simulink model "ThreeL_PWM_direct_2018b"  (R2018b)
settings: Solver=VariableStepAuto  StartTime=0.0  StopTime=0.05  RelTol=1e-3
InitFcn:
  | f_pwm_clk=100e6;
  | T_pwm_clk=1/f_pwm_clk;
libraries: hdlsllib x1
settings Model: Creator=BHK  LastModifiedBy=ga92wum
settings OptimizationCC: BlockReduction=off  ConditionallyExecuteInputs=off  DefaultParameterBehavior=Inlined
settings DebuggingCC: AlgebraicLoopMsg=error
settings HardwareCC: ProdBitPerPointer=32  ProdBitPerSizeT=32  ProdBitPerPtrDiffT=32  ProdLargestAtomicFloat=None  ProdIntDivRoundTo=Undefined  ProdEndianess=Unspecified  ProdWordSize=32  ProdHWDeviceType=ASIC/FPGA->ASIC/FPGA  TargetBitPerPointer=64  TargetBitPerSizeT=64  TargetBitPerPtrDiffT=64  TargetLongLongMode=on  TargetIntDivRoundTo=Zero  TargetEndianess=LittleEndian  TargetWordSize=64  TargetHWDeviceType=Custom Processor->MATLAB Host Computer  ProdEqTarget=off
settings SFSimCC: SimUseLocalCustomCode=off
settings RTWCC: RTWUseLocalCustomCode=off

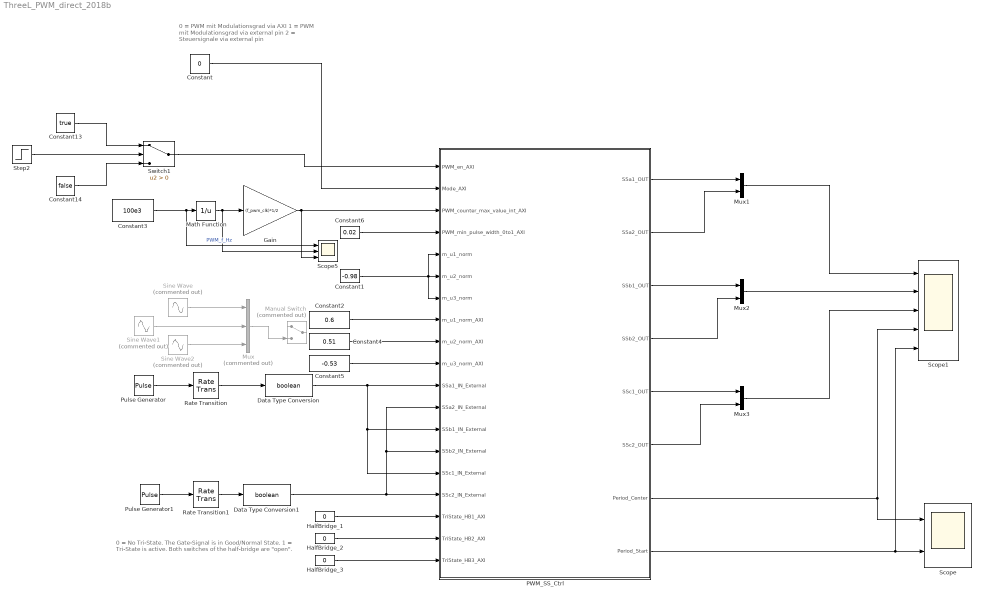
== system ThreeL_PWM_direct_2018b ==
  note: 0 = PWM mit Modulationsgrad via AXI
      | 1 = PWM mit Modulationsgrad via external pin
      | 2 = Steuersignale via external pin
  note: 0 = No Tri-State. The Gate-Signal is in Good/Normal State.
      | 1 = Tri-State is active. Both switches of the half-bridge are "open".
  Constant : Constant  Value=0  OutDataTypeStr=fixdt(0,2,0)  SampleTime=T_pwm_clk
  Constant1 : Constant  Value=-0.98  OutDataTypeStr=fixdt(1,14,12)  SampleTime=T_pwm_clk
  Constant13 : Constant  Value=true  SampleTime=T_pwm_clk
  Constant14 : Constant  Value=false  SampleTime=T_pwm_clk
  Constant2 : Constant  Value=0.6  OutDataTypeStr=fixdt(1,14,12)  SampleTime=T_pwm_clk
  Constant3 : Constant  Value=100e3  OutDataTypeStr=double  SampleTime=T_pwm_clk
  Constant4 : Constant  Value=0.51  OutDataTypeStr=fixdt(1,14,12)  SampleTime=T_pwm_clk
  Constant5 : Constant  Value=-0.53  OutDataTypeStr=fixdt(1,14,12)  SampleTime=T_pwm_clk
  Constant6 : Constant  Value=0.02  OutDataTypeStr=fixdt(1,14,12)  SampleTime=T_pwm_clk
  Data Type Conversion : DataTypeConversion  OutDataTypeStr=boolean
  Data Type Conversion1 : DataTypeConversion  OutDataTypeStr=boolean
  Gain : Gain  Gain=(f_pwm_clk)*1/2  OutDataTypeStr=fixdt(0,20,0)
  HalfBridge_1 : Constant  Value=0  OutDataTypeStr=fixdt(0,2,0)  SampleTime=T_pwm_clk
  HalfBridge_2 : Constant  Value=0  OutDataTypeStr=fixdt(0,2,0)  SampleTime=T_pwm_clk
  HalfBridge_3 : Constant  Value=0  OutDataTypeStr=fixdt(0,2,0)  SampleTime=T_pwm_clk
  Manual Switch : ManualSwitch  Commented=on
  Math Function : Math  Operator=reciprocal  SaturateOnIntegerOverflow=on
  Mux : Mux  Commented=on  Inputs=3
  Mux1 : Mux  Inputs=2
  Mux2 : Mux  Inputs=2
  Mux3 : Mux  Inputs=2
  PWM_SS_Ctrl : Subsystem  TreatAsAtomicUnit=on
  Pulse Generator : DiscretePulseGenerator  PulseType=Time based  Period=2.8e-5  PulseWidth=50  PhaseDelay=0.002
  Pulse Generator1 : DiscretePulseGenerator  PulseType=Time based  Period=2.8e-5  PulseWidth=50  PhaseDelay=0.002
  Rate Transition : RateTransition  OutPortSampleTime=T_pwm_clk
  Rate Transition1 : RateTransition  OutPortSampleTime=T_pwm_clk
  Scope : Scope  NumInputPorts=2
  Scope1 : Scope  NumInputPorts=5
  Scope5 : Scope  NumInputPorts=3
  Sine Wave : Sin  Commented=on  Amplitude=0.8  Frequency=100*pi  Phase=-0.2*pi  SampleTime=T_pwm_clk
  Sine Wave1 : Sin  Commented=on  Amplitude=0.8  Frequency=100*pi  Phase=-0.2*pi + 2/3 * pi  SampleTime=T_pwm_clk
  Sine Wave2 : Sin  Commented=on  Amplitude=0.8  Frequency=100*pi + 4/3 * pi  Phase=-0.2*pi  SampleTime=T_pwm_clk
  Step2 : Step  Time=0.002  SampleTime=T_pwm_clk
  Switch1 : Switch  Criteria=u2 > Threshold
  wires:
  Step2/1 -> Switch1/2
  Constant13/1 -> Switch1/1
  Constant14/1 -> Switch1/3
  Switch1/1 -> PWM_SS_Ctrl/1(PWM_en_AXI)
  Constant/1 -> PWM_SS_Ctrl/2(Mode_AXI)
  Constant6/1 -> PWM_SS_Ctrl/4(PWM_min_pulse_width_0to1_AXI)
  Constant1/1 -> PWM_SS_Ctrl/6(m_u2_norm), PWM_SS_Ctrl/5(m_u1_norm), PWM_SS_Ctrl/7(m_u3_norm)
  Constant3/1 -> Scope5/1, Math Function/1  "PWM_f_Hz"
  Rate Transition/1 -> Data Type Conversion/1
  Pulse Generator/1 -> Rate Transition/1
  HalfBridge_3/1 -> PWM_SS_Ctrl/19(TriState_HB3_AXI)
  HalfBridge_2/1 -> PWM_SS_Ctrl/18(TriState_HB2_AXI)
  HalfBridge_1/1 -> PWM_SS_Ctrl/17(TriState_HB1_AXI)
  Constant2/1 -> PWM_SS_Ctrl/8(m_u1_norm_AXI)
  Mux/1 -> Manual Switch/2
  Sine Wave/1 -> Mux/1
  Sine Wave1/1 -> Mux/2
  Sine Wave2/1 -> Mux/3
  PWM_SS_Ctrl/7(Period_Center) -> Scope1/4, Scope/1
  PWM_SS_Ctrl/8(Period_Start) -> Scope1/5, Scope/2
  Data Type Conversion/1 -> PWM_SS_Ctrl/13(SSb1_IN_External), PWM_SS_Ctrl/15(SSc1_IN_External), PWM_SS_Ctrl/11(SSa1_IN_External)
  Pulse Generator1/1 -> Rate Transition1/1
  Constant4/1 -> PWM_SS_Ctrl/9(m_u2_norm_AXI)
  Constant5/1 -> PWM_SS_Ctrl/10(m_u3_norm_AXI)
  Rate Transition1/1 -> Data Type Conversion1/1
  Data Type Conversion1/1 -> PWM_SS_Ctrl/14(SSb2_IN_External), PWM_SS_Ctrl/12(SSa2_IN_External), PWM_SS_Ctrl/16(SSc2_IN_External)
  PWM_SS_Ctrl/1(SSa1_OUT) -> Mux1/1
  PWM_SS_Ctrl/2(SSa2_OUT) -> Mux1/2
  Mux1/1 -> Scope1/1
  Mux2/1 -> Scope1/2
  PWM_SS_Ctrl/3(SSb1_OUT) -> Mux2/1
  PWM_SS_Ctrl/4(SSb2_OUT) -> Mux2/2
  Mux3/1 -> Scope1/3
  PWM_SS_Ctrl/5(SSc1_OUT) -> Mux3/1
  PWM_SS_Ctrl/6(SSc2_OUT) -> Mux3/2
  Gain/1 -> PWM_SS_Ctrl/3(PWM_counter_max_value_int_AXI), Scope5/3
  Math Function/1 -> Scope5/2, Gain/1

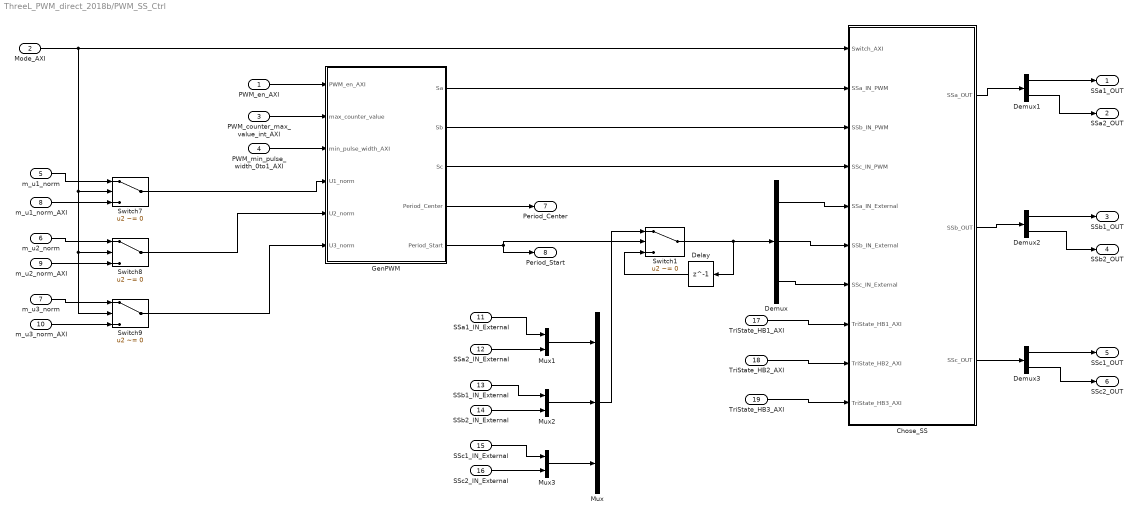
== system ThreeL_PWM_direct_2018b/PWM_SS_Ctrl ==
  PWM_en_AXI : Inport
  Mode_AXI : Inport  Port=2
  PWM_counter_max_value_int_AXI : Inport  Port=3
  PWM_min_pulse_width_0to1_AXI : Inport  Port=4
  m_u1_norm : Inport  Port=5
  m_u2_norm : Inport  Port=6
  m_u3_norm : Inport  Port=7
  m_u1_norm_AXI : Inport  Port=8
  m_u2_norm_AXI : Inport  Port=9
  m_u3_norm_AXI : Inport  Port=10
  SSa1_IN_External : Inport  Port=11
  SSa2_IN_External : Inport  Port=12
  SSb1_IN_External : Inport  Port=13
  SSb2_IN_External : Inport  Port=14
  SSc1_IN_External : Inport  Port=15
  SSc2_IN_External : Inport  Port=16
  TriState_HB1_AXI : Inport  Port=17
  TriState_HB2_AXI : Inport  Port=18
  TriState_HB3_AXI : Inport  Port=19
  Chose_SS : Subsystem
  Delay : Delay  DelayLength=1
  Demux : Demux  Outputs=3
  Demux1 : Demux  Outputs=2
  Demux2 : Demux  Outputs=2
  Demux3 : Demux  Outputs=2
  GenPWM : Subsystem  TreatAsAtomicUnit=on
  Mux : Mux  Inputs=3
  Mux1 : Mux  Inputs=2
  Mux2 : Mux  Inputs=2
  Mux3 : Mux  Inputs=2
  Switch{1,7..9} (4 alike) : Switch  Criteria=u2 ~= 0
  SSa1_OUT : Outport  VectorParamsAs1DForOutWhenUnconnected=off
  SSa2_OUT : Outport  Port=2  VectorParamsAs1DForOutWhenUnconnected=off
  SSb1_OUT : Outport  Port=3  VectorParamsAs1DForOutWhenUnconnected=off
  SSb2_OUT : Outport  Port=4  VectorParamsAs1DForOutWhenUnconnected=off
  SSc1_OUT : Outport  Port=5  VectorParamsAs1DForOutWhenUnconnected=off
  SSc2_OUT : Outport  Port=6  VectorParamsAs1DForOutWhenUnconnected=off
  Period_Center : Outport  Port=7  VectorParamsAs1DForOutWhenUnconnected=off
  Period_Start : Outport  Port=8  VectorParamsAs1DForOutWhenUnconnected=off
  wires:
  PWM_en_AXI/1 -> GenPWM/1(PWM_en_AXI)
  PWM_min_pulse_width_0to1_AXI/1 -> GenPWM/3(min_pulse_width_AXI)
  Switch9/1 -> GenPWM/6(U3_norm)
  m_u1_norm_AXI/1 -> Switch7/3
  m_u1_norm/1 -> Switch7/1
  m_u2_norm/1 -> Switch8/1
  m_u2_norm_AXI/1 -> Switch8/3
  m_u3_norm/1 -> Switch9/1
  m_u3_norm_AXI/1 -> Switch9/3
  Switch8/1 -> GenPWM/5(U2_norm)
  Switch7/1 -> GenPWM/4(U1_norm)
  PWM_counter_max_value_int_AXI/1 -> GenPWM/2(max_counter_value)
  TriState_HB1_AXI/1 -> Chose_SS/8(TriState_HB1_AXI)
  TriState_HB2_AXI/1 -> Chose_SS/9(TriState_HB2_AXI)
  TriState_HB3_AXI/1 -> Chose_SS/10(TriState_HB3_AXI)
  GenPWM/1(Sa) -> Chose_SS/2(SSa_IN_PWM)
  GenPWM/2(Sb) -> Chose_SS/3(SSb_IN_PWM)
  GenPWM/3(Sc) -> Chose_SS/4(SSc_IN_PWM)
  Mode_AXI/1 -> Switch9/2, Switch8/2, Switch7/2, Chose_SS/1(Switch_AXI)
  GenPWM/4(Period_Center) -> Period_Center/1
  Switch1/1 -> Delay/1, Demux/1
  GenPWM/5(Period_Start) -> Switch1/2, Period_Start/1
  Delay/1 -> Switch1/3
  Mux/1 -> Switch1/1
  Demux/1 -> Chose_SS/5(SSa_IN_External)
  Demux/2 -> Chose_SS/6(SSb_IN_External)
  Demux/3 -> Chose_SS/7(SSc_IN_External)
  SSa2_IN_External/1 -> Mux1/2
  SSa1_IN_External/1 -> Mux1/1
  Mux1/1 -> Mux/1
  Mux2/1 -> Mux/2
  SSb1_IN_External/1 -> Mux2/1
  SSb2_IN_External/1 -> Mux2/2
  Mux3/1 -> Mux/3
  SSc1_IN_External/1 -> Mux3/1
  SSc2_IN_External/1 -> Mux3/2
  Chose_SS/1(SSa_OUT) -> Demux1/1
  Chose_SS/2(SSb_OUT) -> Demux2/1
  Chose_SS/3(SSc_OUT) -> Demux3/1
  Demux1/1 -> SSa1_OUT/1
  Demux1/2 -> SSa2_OUT/1
  Demux2/1 -> SSb1_OUT/1
  Demux2/2 -> SSb2_OUT/1
  Demux3/1 -> SSc1_OUT/1
  Demux3/2 -> SSc2_OUT/1

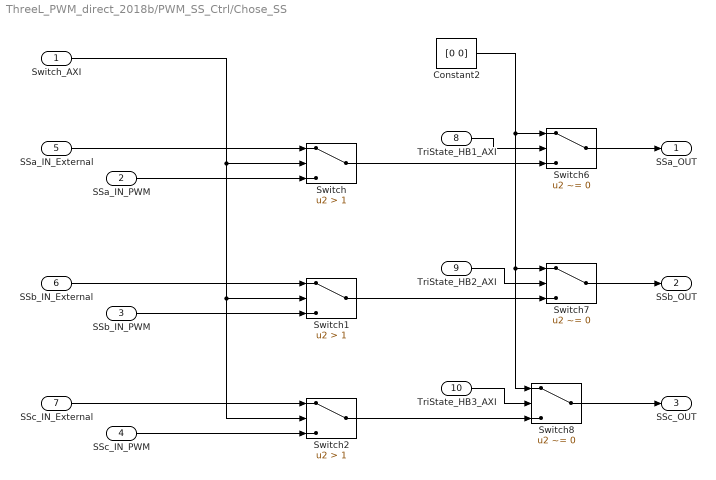
== system ThreeL_PWM_direct_2018b/PWM_SS_Ctrl/Chose_SS ==
  Switch_AXI : Inport
  SSa_IN_PWM : Inport  Port=2
  SSb_IN_PWM : Inport  Port=3
  SSc_IN_PWM : Inport  Port=4
  SSa_IN_External : Inport  Port=5
  SSb_IN_External : Inport  Port=6
  SSc_IN_External : Inport  Port=7
  TriState_HB1_AXI : Inport  Port=8
  TriState_HB2_AXI : Inport  Port=9
  TriState_HB3_AXI : Inport  Port=10
  Constant2 : Constant  Value=[0 0]  OutDataTypeStr=fixdt(0,1,0)  SampleTime=T_pwm_clk
  Switch : Switch  Criteria=u2 > Threshold  Threshold=1
  Switch1 : Switch  Criteria=u2 > Threshold  Threshold=1
  Switch2 : Switch  Criteria=u2 > Threshold  Threshold=1
  Switch6 : Switch  Criteria=u2 ~= 0  Threshold=1
  Switch7 : Switch  Criteria=u2 ~= 0  Threshold=1
  Switch8 : Switch  Criteria=u2 ~= 0  Threshold=1
  SSa_OUT : Outport  VectorParamsAs1DForOutWhenUnconnected=off
  SSb_OUT : Outport  Port=2  VectorParamsAs1DForOutWhenUnconnected=off
  SSc_OUT : Outport  Port=3  VectorParamsAs1DForOutWhenUnconnected=off
  wires:
  Switch_AXI/1 -> Switch2/2, Switch1/2, Switch/2
  Switch/1 -> Switch6/3
  Switch2/1 -> Switch8/3
  Switch1/1 -> Switch7/3
  TriState_HB2_AXI/1 -> Switch7/2
  TriState_HB1_AXI/1 -> Switch6/2
  Constant2/1 -> Switch8/1, Switch7/1, Switch6/1
  SSa_IN_PWM/1 -> Switch/3
  SSb_IN_PWM/1 -> Switch1/3
  SSc_IN_PWM/1 -> Switch2/3
  SSb_IN_External/1 -> Switch1/1
  SSc_IN_External/1 -> Switch2/1
  SSa_IN_External/1 -> Switch/1
  TriState_HB3_AXI/1 -> Switch8/2
  Switch6/1 -> SSa_OUT/1
  Switch7/1 -> SSb_OUT/1
  Switch8/1 -> SSc_OUT/1

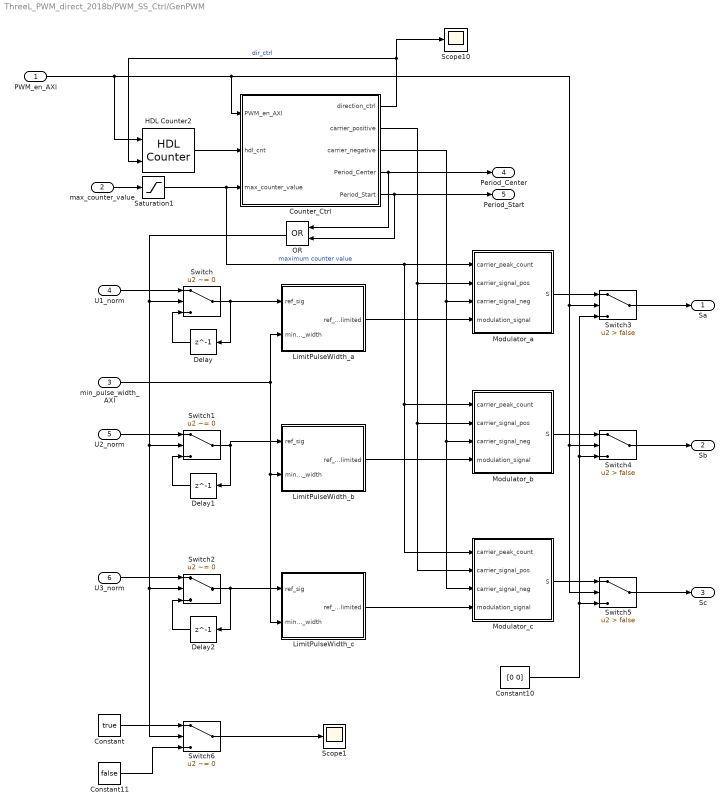
== system ThreeL_PWM_direct_2018b/PWM_SS_Ctrl/GenPWM ==
  PWM_en_AXI : Inport
  max_counter_value : Inport  Port=2
  min_pulse_width_AXI : Inport  Port=3
  U1_norm : Inport  Port=4
  U2_norm : Inport  Port=5
  U3_norm : Inport  Port=6
  Constant : Constant  Value=true  SampleTime=T_pwm_clk
  Constant10 : Constant  Value=[0 0]  OutDataTypeStr=fixdt(0,1,0)  SampleTime=T_pwm_clk
  Constant11 : Constant  Value=false  SampleTime=T_pwm_clk
  Counter_Ctrl : Subsystem
  Delay : Delay  DelayLength=1
  Delay1 : Delay  DelayLength=1
  Delay2 : Delay  DelayLength=1
  HDL Counter2 : hdlsllib/Sources/HDL Counter  CountType=Free running  CountInit=0  CountStep=1  CountMax=100  CountFromType=Initial value  CountFrom=0  CountResetPort=off  CountLoadPort=off  CountEnbPort=on  CountDirPort=on  CountDataType=Unsigned  CountWordLen=20  CountFracLen=0  CountSampTime=1
      settings: SourceProductBaseCode=HD
  LimitPulseWidth_a : Subsystem
  LimitPulseWidth_b : Subsystem
  LimitPulseWidth_c : Subsystem
  Modulator_a : Subsystem
  Modulator_b : Subsystem
  Modulator_c : Subsystem
  OR : Logic  Operator=OR  AllPortsSameDT=off  OutDataTypeStr=boolean
  Saturation1 : Saturate  UpperLimit=10000*50  LowerLimit=10*50
  Scope1 : Scope
  Scope10 : Scope
  Switch{,1..2,6} (4 alike) : Switch  Criteria=u2 ~= 0
  Switch3 : Switch  Criteria=u2 > Threshold  Threshold=false
  Switch4 : Switch  Criteria=u2 > Threshold  Threshold=false
  Switch5 : Switch  Criteria=u2 > Threshold  Threshold=false
  Sa : Outport  VectorParamsAs1DForOutWhenUnconnected=off
  Sb : Outport  Port=2  VectorParamsAs1DForOutWhenUnconnected=off
  Sc : Outport  Port=3  VectorParamsAs1DForOutWhenUnconnected=off
  Period_Center : Outport  Port=4  VectorParamsAs1DForOutWhenUnconnected=off
  Period_Start : Outport  Port=5  VectorParamsAs1DForOutWhenUnconnected=off
  wires:
  Modulator_c/1(S) -> Switch5/1
  PWM_en_AXI/1 -> Counter_Ctrl/1(PWM_en_AXI), Switch3/2, Switch5/2, Switch4/2, HDL Counter2/1
  Modulator_b/1(S) -> Switch4/1
  Constant10/1 -> Switch5/3, Switch4/3, Switch3/3
  Counter_Ctrl/1(direction_ctrl) -> Scope10/1, HDL Counter2/2  "dir_ctrl"
  HDL Counter2/1 -> Counter_Ctrl/2(hdl_cnt)
  Switch/1 -> Delay/1, LimitPulseWidth_a/1(ref_sig)
  Switch1/1 -> LimitPulseWidth_b/1(ref_sig), Delay1/1
  Switch2/1 -> Delay2/1, LimitPulseWidth_c/1(ref_sig)
  max_counter_value/1 -> Saturation1/1
  min_pulse_width_AXI/1 -> LimitPulseWidth_a/2(min_pulse_width), LimitPulseWidth_c/2(min_pulse_width), LimitPulseWidth_b/2(min_pulse_width)
  Modulator_a/1(S) -> Switch3/1
  LimitPulseWidth_a/1(ref_sig_limited) -> Modulator_a/4(modulation_signal)
  Counter_Ctrl/2(carrier_positive) -> Modulator_c/2(carrier_signal_pos), Modulator_b/2(carrier_signal_pos), Modulator_a/2(carrier_signal_pos)
  LimitPulseWidth_c/1(ref_sig_limited) -> Modulator_c/4(modulation_signal)
  Switch3/1 -> Sa/1
  Switch5/1 -> Sc/1
  Switch6/1 -> Scope1/1
  Counter_Ctrl/4(Period_Center) -> OR/1, Period_Center/1
  Switch4/1 -> Sb/1
  Counter_Ctrl/5(Period_Start) -> OR/2, Period_Start/1
  OR/1 -> Switch6/2, Switch2/2, Switch1/2, Switch/2
  U1_norm/1 -> Switch/1
  Delay/1 -> Switch/3
  U2_norm/1 -> Switch1/1
  Delay1/1 -> Switch1/3
  U3_norm/1 -> Switch2/1
  Delay2/1 -> Switch2/3
  Constant/1 -> Switch6/1
  Constant11/1 -> Switch6/3
  Saturation1/1 -> Modulator_b/1(carrier_peak_count), Modulator_c/1(carrier_peak_count), Modulator_a/1(carrier_peak_count), Counter_Ctrl/3(max_counter_value)  "maximum counter value"
  Counter_Ctrl/3(carrier_negative) -> Modulator_b/3(carrier_signal_neg), Modulator_c/3(carrier_signal_neg), Modulator_a/3(carrier_signal_neg)
  LimitPulseWidth_b/1(ref_sig_limited) -> Modulator_b/4(modulation_signal)

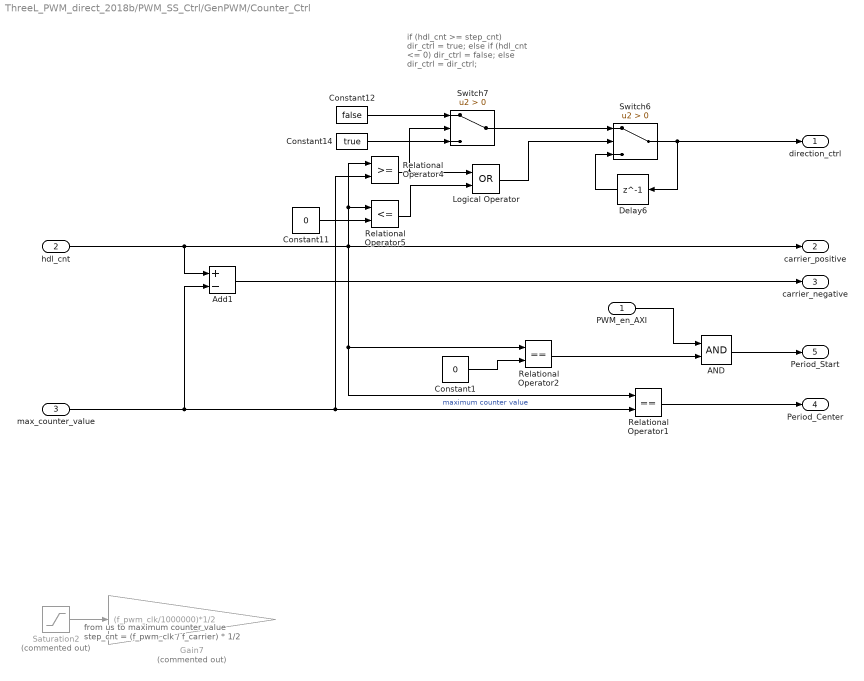
== system ThreeL_PWM_direct_2018b/PWM_SS_Ctrl/GenPWM/Counter_Ctrl ==
  note: if (hdl_cnt >= step_cnt)
      | 	dir_ctrl = true;
      | else if (hdl_cnt <= 0)
      | 	dir_ctrl = false;
      | else
      | 	dir_ctrl = dir_ctrl;
  note: from us to maximum counter value
      | step_cnt = (f_pwm_clk / f_carrier) * 1/2
  PWM_en_AXI : Inport
  hdl_cnt : Inport  Port=2
  max_counter_value : Inport  Port=3
  AND : Logic  AllPortsSameDT=off  OutDataTypeStr=boolean
  Add1 : Sum  Inputs=+-  OutDataTypeStr=fixdt(1,21,0)
  Constant1 : Constant  Value=0  OutDataTypeStr=fixdt(0,20,0)  SampleTime=T_pwm_clk
  Constant11 : Constant  Value=0  OutDataTypeStr=fixdt(0,20,0)  SampleTime=T_pwm_clk
  Constant12 : Constant  Value=false  SampleTime=T_pwm_clk
  Constant14 : Constant  Value=true  SampleTime=T_pwm_clk
  Delay6 : Delay  DelayLength=1
  Gain7 : Gain  Commented=on  Gain=(f_pwm_clk/1000000)*1/2  OutDataTypeStr=fixdt(0,20,0)
  Logical Operator : Logic  Operator=OR  AllPortsSameDT=off  OutDataTypeStr=boolean
  Relational Operator1 : RelationalOperator  Operator===  OutDataTypeStr=boolean  RndMeth=Nearest
  Relational Operator2 : RelationalOperator  Operator===  OutDataTypeStr=boolean  RndMeth=Nearest
  Relational Operator4 : RelationalOperator  OutDataTypeStr=boolean  RndMeth=Nearest
  Relational Operator5 : RelationalOperator  Operator=<=  OutDataTypeStr=boolean  RndMeth=Nearest
  Saturation2 : Saturate  Commented=on  UpperLimit=10000  LowerLimit=10
  Switch6 : Switch  Criteria=u2 > Threshold
  Switch7 : Switch  Criteria=u2 > Threshold
  direction_ctrl : Outport  VectorParamsAs1DForOutWhenUnconnected=off
  carrier_positive : Outport  Port=2  VectorParamsAs1DForOutWhenUnconnected=off
  carrier_negative : Outport  Port=3  VectorParamsAs1DForOutWhenUnconnected=off
  Period_Center : Outport  Port=4  VectorParamsAs1DForOutWhenUnconnected=off
  Period_Start : Outport  Port=5  VectorParamsAs1DForOutWhenUnconnected=off
  wires:
  Switch6/1 -> Delay6/1, direction_ctrl/1
  Relational Operator4/1 -> Switch7/2, Logical Operator/1
  Relational Operator5/1 -> Logical Operator/2
  Constant11/1 -> Relational Operator5/2
  Logical Operator/1 -> Switch6/2
  Switch7/1 -> Switch6/1
  Constant12/1 -> Switch7/1
  Constant14/1 -> Switch7/3
  Delay6/1 -> Switch6/3
  max_counter_value/1 -> Add1/2, Relational Operator1/2, Relational Operator4/2  "maximum counter value"
  hdl_cnt/1 -> Add1/1, Relational Operator5/1, Relational Operator4/1, Relational Operator2/1, Relational Operator1/1, carrier_positive/1
  Relational Operator1/1 -> Period_Center/1
  Constant1/1 -> Relational Operator2/2
  AND/1 -> Period_Start/1
  Relational Operator2/1 -> AND/2
  PWM_en_AXI/1 -> AND/1
  Saturation2/1 -> Gain7/1
  Add1/1 -> carrier_negative/1

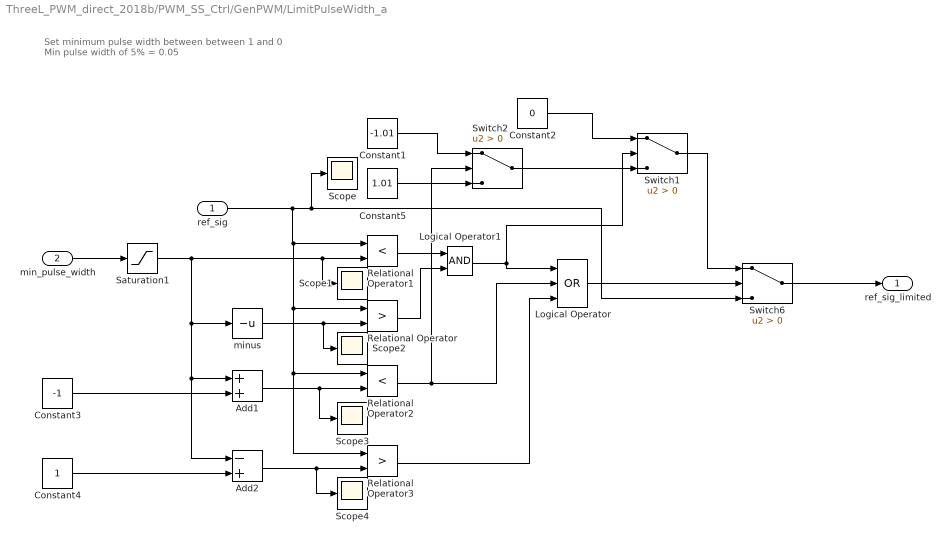
== system ThreeL_PWM_direct_2018b/PWM_SS_Ctrl/GenPWM/LimitPulseWidth_a ==
  note: Set minimum pulse width between between 1 and 0
      | Min pulse width of 5% = 0.05
  ref_sig : Inport
  min_pulse_width : Inport  Port=2
  Add1 : Sum  OutDataTypeStr=fixdt(1,14,12)
  Add2 : Sum  Inputs=-+  OutDataTypeStr=fixdt(1,14,12)
  Constant1 : Constant  Value=-1.01  OutDataTypeStr=fixdt(1,14,12)  SampleTime=T_pwm_clk
  Constant2 : Constant  Value=0  OutDataTypeStr=fixdt(1,14,12)  SampleTime=T_pwm_clk
  Constant3 : Constant  Value=-1  OutDataTypeStr=fixdt(1,14,12)  SampleTime=T_pwm_clk
  Constant4 : Constant  OutDataTypeStr=fixdt(1,14,12)  SampleTime=T_pwm_clk
  Constant5 : Constant  Value=1.01  OutDataTypeStr=fixdt(1,14,12)  SampleTime=T_pwm_clk
  Logical Operator : Logic  Operator=OR  Inputs=3  AllPortsSameDT=off  OutDataTypeStr=boolean
  Logical Operator1 : Logic  AllPortsSameDT=off  OutDataTypeStr=boolean
  Relational Operator : RelationalOperator  Operator=>  OutDataTypeStr=boolean  RndMeth=Nearest
  Relational Operator1 : RelationalOperator  Operator=<  OutDataTypeStr=boolean  RndMeth=Nearest
  Relational Operator2 : RelationalOperator  Operator=<  OutDataTypeStr=boolean  RndMeth=Nearest
  Relational Operator3 : RelationalOperator  Operator=>  OutDataTypeStr=boolean  RndMeth=Nearest
  Saturation1 : Saturate  UpperLimit=1  LowerLimit=0  OutDataTypeStr=fixdt(1,14,12)
  Scope{,1..4} (5 alike) : Scope
  Switch1 : Switch  Criteria=u2 > Threshold
  Switch2 : Switch  Criteria=u2 > Threshold
  Switch6 : Switch  Criteria=u2 > Threshold
  minus : UnaryMinus
  ref_sig_limited : Outport  VectorParamsAs1DForOutWhenUnconnected=off
  wires:
  Constant3/1 -> Add1/2
  Add2/1 -> Scope4/1, Relational Operator3/2
  ref_sig/1 -> Relational Operator2/1, Relational Operator3/1, Relational Operator/1, Relational Operator1/1, Scope/1, Switch6/3
  Relational Operator/1 -> Logical Operator1/2
  Switch1/1 -> Switch6/1
  Constant4/1 -> Add2/2
  minus/1 -> Scope2/1, Relational Operator/2
  Switch2/1 -> Switch1/3
  Logical Operator/1 -> Switch6/2
  Constant1/1 -> Switch2/1
  Constant5/1 -> Switch2/3
  Relational Operator1/1 -> Logical Operator1/1
  Relational Operator3/1 -> Logical Operator/3
  Add1/1 -> Scope3/1, Relational Operator2/2
  Saturation1/1 -> Scope1/1, Relational Operator1/2, minus/1, Add2/1, Add1/1
  Switch6/1 -> ref_sig_limited/1
  Relational Operator2/1 -> Switch2/2, Logical Operator/2
  Logical Operator1/1 -> Logical Operator/1, Switch1/2
  min_pulse_width/1 -> Saturation1/1
  Constant2/1 -> Switch1/1

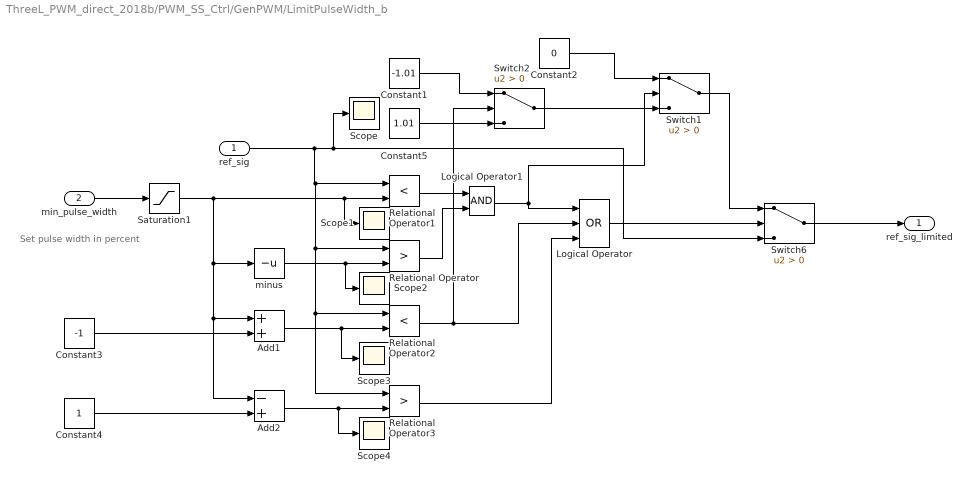
== system ThreeL_PWM_direct_2018b/PWM_SS_Ctrl/GenPWM/LimitPulseWidth_b ==
  note: Set pulse width in percent
  ref_sig : Inport
  min_pulse_width : Inport  Port=2
  Add1 : Sum  OutDataTypeStr=fixdt(1,14,12)
  Add2 : Sum  Inputs=-+  OutDataTypeStr=fixdt(1,14,12)
  Constant1 : Constant  Value=-1.01  OutDataTypeStr=fixdt(1,14,12)  SampleTime=T_pwm_clk
  Constant2 : Constant  Value=0  OutDataTypeStr=fixdt(1,14,12)  SampleTime=T_pwm_clk
  Constant3 : Constant  Value=-1  OutDataTypeStr=fixdt(1,14,12)  SampleTime=T_pwm_clk
  Constant4 : Constant  OutDataTypeStr=fixdt(1,14,12)  SampleTime=T_pwm_clk
  Constant5 : Constant  Value=1.01  OutDataTypeStr=fixdt(1,14,12)  SampleTime=T_pwm_clk
  Logical Operator : Logic  Operator=OR  Inputs=3  AllPortsSameDT=off  OutDataTypeStr=boolean
  Logical Operator1 : Logic  AllPortsSameDT=off  OutDataTypeStr=boolean
  Relational Operator : RelationalOperator  Operator=>  OutDataTypeStr=boolean  RndMeth=Nearest
  Relational Operator1 : RelationalOperator  Operator=<  OutDataTypeStr=boolean  RndMeth=Nearest
  Relational Operator2 : RelationalOperator  Operator=<  OutDataTypeStr=boolean  RndMeth=Nearest
  Relational Operator3 : RelationalOperator  Operator=>  OutDataTypeStr=boolean  RndMeth=Nearest
  Saturation1 : Saturate  UpperLimit=1  LowerLimit=0  OutDataTypeStr=fixdt(1,14,12)
  Scope{,1..4} (5 alike) : Scope
  Switch1 : Switch  Criteria=u2 > Threshold
  Switch2 : Switch  Criteria=u2 > Threshold
  Switch6 : Switch  Criteria=u2 > Threshold
  minus : UnaryMinus
  ref_sig_limited : Outport  VectorParamsAs1DForOutWhenUnconnected=off
  wires:
  Constant3/1 -> Add1/2
  Add2/1 -> Scope4/1, Relational Operator3/2
  ref_sig/1 -> Relational Operator2/1, Relational Operator3/1, Relational Operator/1, Relational Operator1/1, Scope/1, Switch6/3
  Relational Operator/1 -> Logical Operator1/2
  Switch1/1 -> Switch6/1
  Constant4/1 -> Add2/2
  minus/1 -> Scope2/1, Relational Operator/2
  Switch2/1 -> Switch1/3
  Logical Operator/1 -> Switch6/2
  Constant1/1 -> Switch2/1
  Constant5/1 -> Switch2/3
  Relational Operator1/1 -> Logical Operator1/1
  Relational Operator3/1 -> Logical Operator/3
  Add1/1 -> Scope3/1, Relational Operator2/2
  Saturation1/1 -> Scope1/1, Relational Operator1/2, minus/1, Add2/1, Add1/1
  Switch6/1 -> ref_sig_limited/1
  Relational Operator2/1 -> Switch2/2, Logical Operator/2
  Logical Operator1/1 -> Logical Operator/1, Switch1/2
  min_pulse_width/1 -> Saturation1/1
  Constant2/1 -> Switch1/1

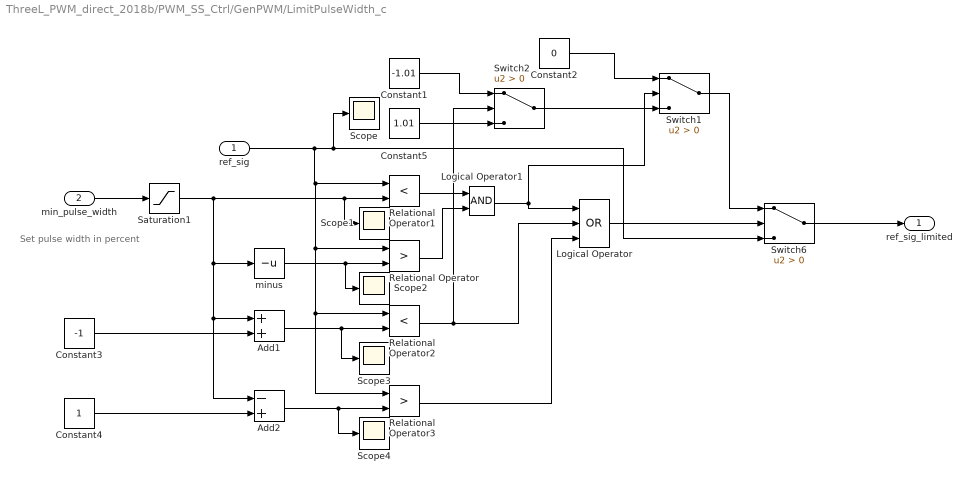
== system ThreeL_PWM_direct_2018b/PWM_SS_Ctrl/GenPWM/LimitPulseWidth_c ==
  note: Set pulse width in percent
  ref_sig : Inport
  min_pulse_width : Inport  Port=2
  Add1 : Sum  OutDataTypeStr=fixdt(1,14,12)
  Add2 : Sum  Inputs=-+  OutDataTypeStr=fixdt(1,14,12)
  Constant1 : Constant  Value=-1.01  OutDataTypeStr=fixdt(1,14,12)  SampleTime=T_pwm_clk
  Constant2 : Constant  Value=0  OutDataTypeStr=fixdt(1,14,12)  SampleTime=T_pwm_clk
  Constant3 : Constant  Value=-1  OutDataTypeStr=fixdt(1,14,12)  SampleTime=T_pwm_clk
  Constant4 : Constant  OutDataTypeStr=fixdt(1,14,12)  SampleTime=T_pwm_clk
  Constant5 : Constant  Value=1.01  OutDataTypeStr=fixdt(1,14,12)  SampleTime=T_pwm_clk
  Logical Operator : Logic  Operator=OR  Inputs=3  AllPortsSameDT=off  OutDataTypeStr=boolean
  Logical Operator1 : Logic  AllPortsSameDT=off  OutDataTypeStr=boolean
  Relational Operator : RelationalOperator  Operator=>  OutDataTypeStr=boolean  RndMeth=Nearest
  Relational Operator1 : RelationalOperator  Operator=<  OutDataTypeStr=boolean  RndMeth=Nearest
  Relational Operator2 : RelationalOperator  Operator=<  OutDataTypeStr=boolean  RndMeth=Nearest
  Relational Operator3 : RelationalOperator  Operator=>  OutDataTypeStr=boolean  RndMeth=Nearest
  Saturation1 : Saturate  UpperLimit=1  LowerLimit=0  OutDataTypeStr=fixdt(1,14,12)
  Scope{,1..4} (5 alike) : Scope
  Switch1 : Switch  Criteria=u2 > Threshold
  Switch2 : Switch  Criteria=u2 > Threshold
  Switch6 : Switch  Criteria=u2 > Threshold
  minus : UnaryMinus
  ref_sig_limited : Outport  VectorParamsAs1DForOutWhenUnconnected=off
  wires:
  Constant3/1 -> Add1/2
  Add2/1 -> Scope4/1, Relational Operator3/2
  ref_sig/1 -> Relational Operator2/1, Relational Operator3/1, Relational Operator/1, Relational Operator1/1, Scope/1, Switch6/3
  Relational Operator/1 -> Logical Operator1/2
  Switch1/1 -> Switch6/1
  Constant4/1 -> Add2/2
  minus/1 -> Scope2/1, Relational Operator/2
  Switch2/1 -> Switch1/3
  Logical Operator/1 -> Switch6/2
  Constant1/1 -> Switch2/1
  Constant5/1 -> Switch2/3
  Relational Operator1/1 -> Logical Operator1/1
  Relational Operator3/1 -> Logical Operator/3
  Add1/1 -> Scope3/1, Relational Operator2/2
  Saturation1/1 -> Scope1/1, Relational Operator1/2, minus/1, Add2/1, Add1/1
  Switch6/1 -> ref_sig_limited/1
  Relational Operator2/1 -> Switch2/2, Logical Operator/2
  Logical Operator1/1 -> Logical Operator/1, Switch1/2
  min_pulse_width/1 -> Saturation1/1
  Constant2/1 -> Switch1/1

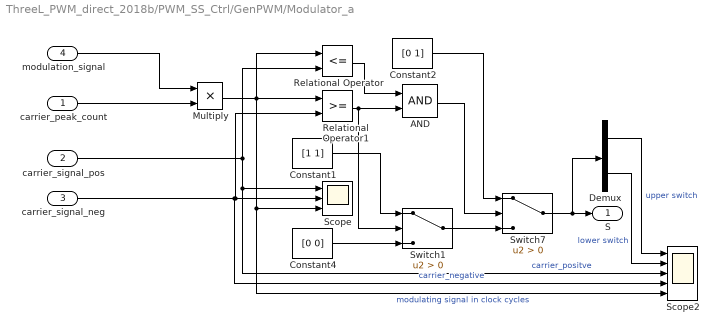
== system ThreeL_PWM_direct_2018b/PWM_SS_Ctrl/GenPWM/Modulator_a ==
  carrier_peak_count : Inport  OutDataTypeStr=fixdt(0,20,0)
  carrier_signal_pos : Inport  Port=2  OutDataTypeStr=fixdt(0,20,0)
  carrier_signal_neg : Inport  Port=3  OutDataTypeStr=fixdt(1,21,0)
  modulation_signal : Inport  Port=4  OutDataTypeStr=fixdt(1,14,12)
  AND : Logic  AllPortsSameDT=off  OutDataTypeStr=boolean
  Constant1 : Constant  Value=[1 1]  OutDataTypeStr=fixdt(0,1,0)  SampleTime=T_pwm_clk
  Constant2 : Constant  Value=[0 1]  OutDataTypeStr=fixdt(0,1,0)  SampleTime=T_pwm_clk
  Constant4 : Constant  Value=[0 0]  OutDataTypeStr=fixdt(0,1,0)  SampleTime=T_pwm_clk
  Demux : Demux  Outputs=2
  Multiply : Product  OutDataTypeStr=fixdt(1,21,0)
  Relational Operator : RelationalOperator  Operator=<=  OutDataTypeStr=boolean  RndMeth=Nearest
  Relational Operator1 : RelationalOperator  OutDataTypeStr=boolean  RndMeth=Nearest
  Scope : Scope  NumInputPorts=3
  Scope2 : Scope  NumInputPorts=5
  Switch1 : Switch  Criteria=u2 > Threshold
  Switch7 : Switch  Criteria=u2 > Threshold
  S : Outport  VectorParamsAs1DForOutWhenUnconnected=off
  wires:
  Constant1/1 -> Switch1/1
  Demux/1 -> Scope2/1  "upper switch"
  Relational Operator/1 -> AND/1
  carrier_signal_neg/1 -> Relational Operator1/2, Scope/2, Scope2/4  "carrier_negative"
  Constant4/1 -> Switch1/3
  carrier_peak_count/1 -> Multiply/2
  Demux/2 -> Scope2/2  "lower switch"
  AND/1 -> Switch7/2
  Constant2/1 -> Switch7/1
  modulation_signal/1 -> Multiply/1
  Switch1/1 -> Switch7/3
  carrier_signal_pos/1 -> Relational Operator/2, Scope/1, Scope2/3  "carrier_positve"
  Multiply/1 -> Relational Operator1/1, Relational Operator/1, Scope2/5, Scope/3  "modulating signal in clock cycles"
  Relational Operator1/1 -> AND/2, Switch1/2
  Switch7/1 -> S/1, Demux/1

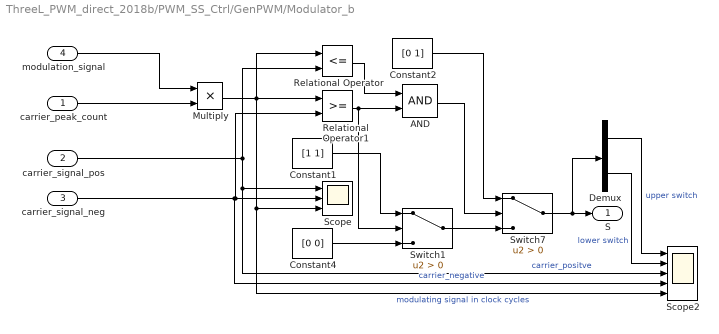
== system ThreeL_PWM_direct_2018b/PWM_SS_Ctrl/GenPWM/Modulator_b ==
  carrier_peak_count : Inport  OutDataTypeStr=fixdt(0,20,0)
  carrier_signal_pos : Inport  Port=2  OutDataTypeStr=fixdt(0,20,0)
  carrier_signal_neg : Inport  Port=3  OutDataTypeStr=fixdt(1,21,0)
  modulation_signal : Inport  Port=4  OutDataTypeStr=fixdt(1,14,12)
  AND : Logic  AllPortsSameDT=off  OutDataTypeStr=boolean
  Constant1 : Constant  Value=[1 1]  OutDataTypeStr=fixdt(0,1,0)  SampleTime=T_pwm_clk
  Constant2 : Constant  Value=[0 1]  OutDataTypeStr=fixdt(0,1,0)  SampleTime=T_pwm_clk
  Constant4 : Constant  Value=[0 0]  OutDataTypeStr=fixdt(0,1,0)  SampleTime=T_pwm_clk
  Demux : Demux  Outputs=2
  Multiply : Product  OutDataTypeStr=fixdt(1,21,0)
  Relational Operator : RelationalOperator  Operator=<=  OutDataTypeStr=boolean  RndMeth=Nearest
  Relational Operator1 : RelationalOperator  OutDataTypeStr=boolean  RndMeth=Nearest
  Scope : Scope  NumInputPorts=3
  Scope2 : Scope  NumInputPorts=5
  Switch1 : Switch  Criteria=u2 > Threshold
  Switch7 : Switch  Criteria=u2 > Threshold
  S : Outport  VectorParamsAs1DForOutWhenUnconnected=off
  wires:
  Switch7/1 -> Demux/1, S/1
  Relational Operator1/1 -> Switch1/2, AND/2
  Multiply/1 -> Scope/3, Scope2/5, Relational Operator/1, Relational Operator1/1  "modulating signal in clock cycles"
  carrier_signal_pos/1 -> Scope2/3, Scope/1, Relational Operator/2  "carrier_positve"
  Switch1/1 -> Switch7/3
  modulation_signal/1 -> Multiply/1
  Constant2/1 -> Switch7/1
  AND/1 -> Switch7/2
  Demux/2 -> Scope2/2  "lower switch"
  carrier_peak_count/1 -> Multiply/2
  Constant4/1 -> Switch1/3
  carrier_signal_neg/1 -> Scope2/4, Scope/2, Relational Operator1/2  "carrier_negative"
  Relational Operator/1 -> AND/1
  Demux/1 -> Scope2/1  "upper switch"
  Constant1/1 -> Switch1/1

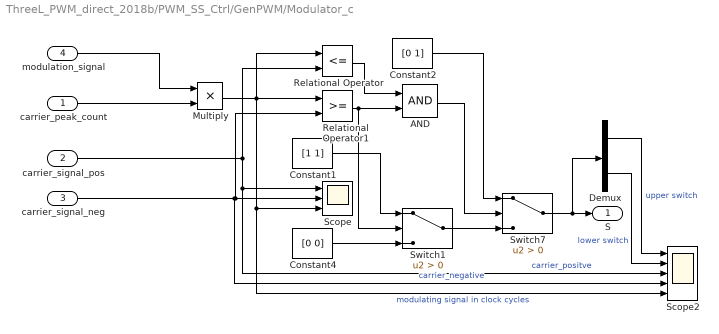
== system ThreeL_PWM_direct_2018b/PWM_SS_Ctrl/GenPWM/Modulator_c ==
  carrier_peak_count : Inport  OutDataTypeStr=fixdt(0,20,0)
  carrier_signal_pos : Inport  Port=2  OutDataTypeStr=fixdt(0,20,0)
  carrier_signal_neg : Inport  Port=3  OutDataTypeStr=fixdt(1,21,0)
  modulation_signal : Inport  Port=4  OutDataTypeStr=fixdt(1,14,12)
  AND : Logic  AllPortsSameDT=off  OutDataTypeStr=boolean
  Constant1 : Constant  Value=[1 1]  OutDataTypeStr=fixdt(0,1,0)  SampleTime=T_pwm_clk
  Constant2 : Constant  Value=[0 1]  OutDataTypeStr=fixdt(0,1,0)  SampleTime=T_pwm_clk
  Constant4 : Constant  Value=[0 0]  OutDataTypeStr=fixdt(0,1,0)  SampleTime=T_pwm_clk
  Demux : Demux  Outputs=2
  Multiply : Product  OutDataTypeStr=fixdt(1,21,0)
  Relational Operator : RelationalOperator  Operator=<=  OutDataTypeStr=boolean  RndMeth=Nearest
  Relational Operator1 : RelationalOperator  OutDataTypeStr=boolean  RndMeth=Nearest
  Scope : Scope  NumInputPorts=3
  Scope2 : Scope  NumInputPorts=5
  Switch1 : Switch  Criteria=u2 > Threshold
  Switch7 : Switch  Criteria=u2 > Threshold
  S : Outport  VectorParamsAs1DForOutWhenUnconnected=off
  wires:
  Constant1/1 -> Switch1/1
  Demux/1 -> Scope2/1  "upper switch"
  Relational Operator/1 -> AND/1
  carrier_signal_neg/1 -> Relational Operator1/2, Scope/2, Scope2/4  "carrier_negative"
  Constant4/1 -> Switch1/3
  carrier_peak_count/1 -> Multiply/2
  Demux/2 -> Scope2/2  "lower switch"
  AND/1 -> Switch7/2
  Constant2/1 -> Switch7/1
  modulation_signal/1 -> Multiply/1
  Switch1/1 -> Switch7/3
  carrier_signal_pos/1 -> Relational Operator/2, Scope/1, Scope2/3  "carrier_positve"
  Multiply/1 -> Relational Operator1/1, Relational Operator/1, Scope2/5, Scope/3  "modulating signal in clock cycles"
  Relational Operator1/1 -> AND/2, Switch1/2
  Switch7/1 -> S/1, Demux/1
